simulink model "SF019B_PwrLimr"  (R2013b)
settings: Solver=VariableStepDiscrete  StartTime=0.0  StopTime=10  RelTol=1e-3
values from neighbouring files (symbols this model uses):
  ARCHGLBPRM_2MILLISEC_SEC_F32 = DataDict.Constant    [SF019B_PwrLimr_DataDict.m]
  ELECGLBPRM_IVTRCNT_CNT_U08 = DataDict.ConfigParam    [SF019B_PwrLimr_DataDict.m]
  PwrLimrBackEmfConStdT = DataDict.Calibration    [SF019B_PwrLimr_DataDict.m]
  PwrLimrBrdgVltgAdjSlew = DataDict.Calibration    [SF019B_PwrLimr_DataDict.m]
  PwrLimrBrdgVltgAltFltAdj = DataDict.Calibration    [SF019B_PwrLimr_DataDict.m]
  PwrLimrFilAssiRednThd = DataDict.Calibration    [SF019B_PwrLimr_DataDict.m]
  PwrLimrLoVoltAssiRcvrThd = DataDict.Calibration    [SF019B_PwrLimr_DataDict.m]
  PwrLimrLoVoltAssiRcvrTi = DataDict.Calibration    [SF019B_PwrLimr_DataDict.m]
  PWRLIMRMILLISECTOSEC_SECPERMILLISEC_F32 = DataDict.Constant    [SF019B_PwrLimr_DataDict.m]
  PwrLimrMotEnvlpX = DataDict.Calibration    [SF019B_PwrLimr_DataDict.m]
  PwrLimrMotEnvlpY = DataDict.Calibration    [SF019B_PwrLimr_DataDict.m]
  PwrLimrSpdAdjSlewDec = DataDict.Calibration    [SF019B_PwrLimr_DataDict.m]
  PwrLimrSpdAdjSlewEna = DataDict.Calibration    [SF019B_PwrLimr_DataDict.m]
  PwrLimrSpdAdjSlewInc = DataDict.Calibration    [SF019B_PwrLimr_DataDict.m]
  PwrLimrStdOperMotEnvlpX = DataDict.Calibration    [SF019B_PwrLimr_DataDict.m]
  PwrLimrStdOperMotEnvlpY = DataDict.Calibration    [SF019B_PwrLimr_DataDict.m]
  PwrLimrVltgDptMotVelOffsX = DataDict.Calibration    [SF019B_PwrLimr_DataDict.m]
  PwrLimrVltgDptMotVelOffsY = DataDict.Calibration    [SF019B_PwrLimr_DataDict.m]
undefined symbols (not defined in the file): ARCHGLBPRM_10MILLISEC_SEC_F32, PwrLimrAssiRednLpFilFrq, PwrLimrMotVelLpFilFrq
libraries: simulink x12, NxtrLim x2
(part 2 of 2)

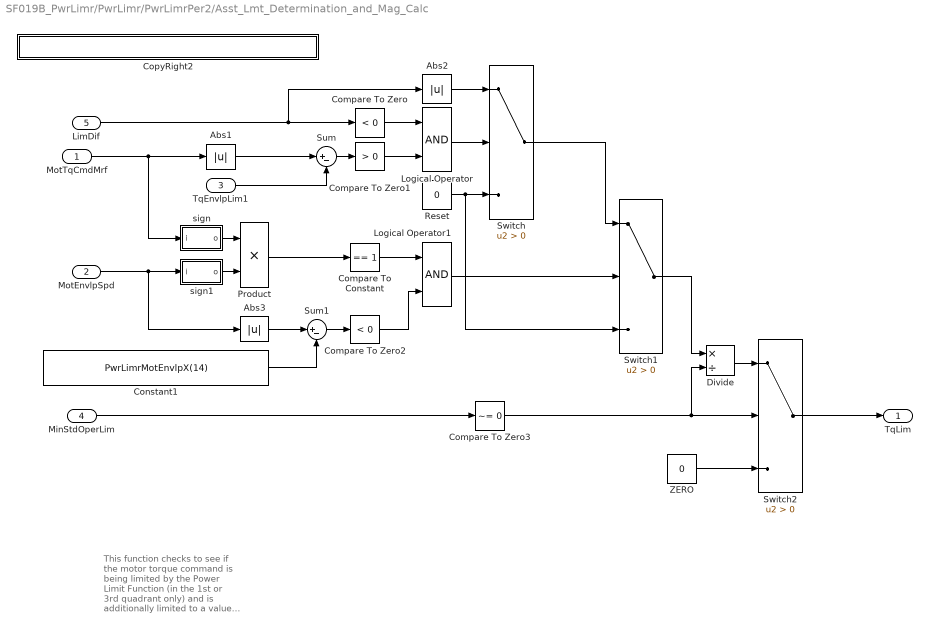
== system SF019B_PwrLimr/PwrLimr/PwrLimrPer2/Asst_Lmt_Determination_and_Mag_Calc ==
  note: This function checks to see if the motor torque command is being limited by the Power Limit Function
      | (in the 1st or 3rd quadrant only) and is additionally limited to a value less than the full performance at
      | the minimum standard operating condition voltage.
      |
      | The magnitude of assist reduction is calculated as the amount of assist reduction divided
      | by full performance in minimum standard operating condition voltage.
  MotTqCmdMrf : Inport
  MotEnvlpSpd : Inport  Port=2
  TqEnvlpLim1 : Inport  Port=3
  MinStdOperLim : Inport  Port=4
  LimDif : Inport  Port=5
  Abs1 : Abs
  Abs2 : Abs
  Abs3 : Abs
  Compare To Constant : simulink/Logic and Bit Operations/Compare To Constant  relop===  const=1  OutDataTypeStr=uint8
  Compare To Zero : simulink/Logic and Bit Operations/Compare To Zero  relop=<  OutDataTypeStr=uint8
  Compare To Zero1 : simulink/Logic and Bit Operations/Compare To Zero  relop=>  OutDataTypeStr=uint8
  Compare To Zero2 : simulink/Logic and Bit Operations/Compare To Zero  relop=<  OutDataTypeStr=uint8
  Compare To Zero3 : simulink/Logic and Bit Operations/Compare To Zero  relop=~=  OutDataTypeStr=uint8
  Constant1 : Constant  Value=PwrLimrMotEnvlpX(14)
  CopyRight2 : Subsystem  Description=|  mask(Copyright Information){none=on}
      | Copyright info block.                                               
      |                                                                     
      | Place copyright information at the top of every subsystem in design.
      mask prompts: none "No parameters"
      mask help: Place copyright information at the top of every subsystem in design.
      mask Display:
      | NxtrConf = 'Nexteer Confidential';
      | 
      | sys = bdroot; %handle for the current model ("system")
      | first = get_param(sys,'Created');
      | first = first(end-3:end);  %year is last four digits
      | 
      | last = get_param(sys,'LastModifiedDate');
      | if isempty(last)
      |     last = datestr(now,'yyyy');
      | else
      |     last = last(end-3:end);
      | end
      | 
      | if strcmp(first,last)
      |     fprintf('%s -- Copyright %s Nexteer',NxtrConf,first)
      | else
      |     fprintf('%s -- %s%s- %s Nexteer',NxtrConf,char(169),first,last)
      | end
  Divide : Product  Inputs=*/
  Logical Operator : Logic  AllPortsSameDT=off  OutDataTypeStr=boolean
  Logical Operator1 : Logic  AllPortsSameDT=off  OutDataTypeStr=boolean
  Product : Product  RndMeth=Zero
  Reset : Constant  Value=0
  Sum : Sum  Inputs=|+-
  Sum1 : Sum  Inputs=|+-
  Switch : Switch  Criteria=u2 > Threshold
  Switch1 : Switch  Criteria=u2 > Threshold
  Switch2 : Switch  Criteria=u2 > Threshold
      settings: AttributesFormatString=Checking for divide-by-zero
  ZERO : Constant  Value=0
  sign : Subsystem  mask(2-state sign){}
      mask help: version: Nov 30, 2012
      mask Help:
      | Input < 0, Output = -1
      | Input = 0, Output = +1
      | Input > 0, Output = +1
      mask Display: disp 'sign'
  sign1 : Subsystem  mask(2-state sign){}
      mask help: version: Nov 30, 2012
      mask Help:
      | Input < 0, Output = -1
      | Input = 0, Output = +1
      | Input > 0, Output = +1
      mask Display: disp 'sign'
  TqLim : Outport
  wires:
  Sum/1 -> Compare To Zero1/1
  Compare To Zero/1 -> Logical Operator/1
  Compare To Zero1/1 -> Logical Operator/2
  Logical Operator/1 -> Switch/2
  Abs2/1 -> Switch/1
  Reset/1 -> Switch/3, Switch1/3
  LimDif/1 -> Compare To Zero/1, Abs2/1
  MotTqCmdMrf/1 -> Abs1/1, sign/1(i)
  TqEnvlpLim1/1 -> Sum/2
  Abs1/1 -> Sum/1
  Switch1/1 -> Divide/1
  MotEnvlpSpd/1 -> Abs3/1, sign1/1(i)
  sign/1(o) -> Product/1
  sign1/1(o) -> Product/2
  Product/1 -> Compare To Constant/1
  Compare To Constant/1 -> Logical Operator1/1
  Switch/1 -> Switch1/1
  Abs3/1 -> Sum1/1
  Constant1/1 -> Sum1/2
  Sum1/1 -> Compare To Zero2/1
  Compare To Zero2/1 -> Logical Operator1/2
  Logical Operator1/1 -> Switch1/2
  MinStdOperLim/1 -> Compare To Zero3/1
  ZERO/1 -> Switch2/3
  Compare To Zero3/1 -> Switch2/2, Divide/2
  Divide/1 -> Switch2/1
  Switch2/1 -> TqLim/1

== system SF019B_PwrLimr/PwrLimr/PwrLimrPer2/CopyRight2 ==

== system SF019B_PwrLimr/PwrLimr/PwrLimrPer1/Battery_Voltage_Fn/CopyRight2 ==

== system SF019B_PwrLimr/PwrLimr/PwrLimrPer1/Max_Mtr_Curr_Lmt_Fn/CopyRight2 ==

== system SF019B_PwrLimr/PwrLimr/PwrLimrPer1/MinStdOp_Volt_Max_Net_Assist/CopyRight2 ==

== system SF019B_PwrLimr/PwrLimr/PwrLimrPer1/OpVel_Offset_Slew_Rate_Lmt/CopyRight2 ==

== system SF019B_PwrLimr/PwrLimr/PwrLimrPer1/Output_Velocity_Fn/Apply_Limit_Else ==
  SignMotEnvlpSpd : Inport
  TqLim1 : Inport  Port=2
  Product2 : Product  RndMeth=Zero
  MRFMtrTrqCmdTemp_MtrNm : Outport
  wires:
  TqLim1/1 -> Product2/2
  SignMotEnvlpSpd/1 -> Product2/1
  Product2/1 -> MRFMtrTrqCmdTemp_MtrNm/1

== system SF019B_PwrLimr/PwrLimr/PwrLimrPer1/Output_Velocity_Fn/Apply_Limit_If ==
  CntDisMtrTrqCmdPerInvMRF : Inport
  SignMotEnvlpSpd : Inport  Port=2
  TqLim1 : Inport  Port=3
  TqLim4 : Inport  Port=4
  Product : Product  RndMeth=Zero
  Product1 : Product  RndMeth=Zero
  Saturation_Dynamic : simulink/Discontinuities/Saturation Dynamic  OutMin=-8.8  OutMax=8.8  OutDataTypeStr=Inherit: Same as second input  OutDataType=fixdt(1, 16)  OutScaling=2^-10  DoSatur=off
  MRFMtrTrqCmdTemp_MtrNm : Outport
  wires:
  Saturation_Dynamic/1 -> Product1/2
  Product/1 -> Saturation_Dynamic/2
  SignMotEnvlpSpd/1 -> Product/1, Product1/1
  TqLim1/1 -> Saturation_Dynamic/1
  Product1/1 -> MRFMtrTrqCmdTemp_MtrNm/1
  CntDisMtrTrqCmdPerInvMRF/1 -> Product/2
  TqLim4/1 -> Saturation_Dynamic/3

== system SF019B_PwrLimr/PwrLimr/PwrLimrPer1/Output_Velocity_Fn/ChooseMax4 ==
  TqEnvlpLim4 : Inport
  TLimMaxCurr : Inport  Port=2
  Gain2 : Gain  Gain=-1
  MinMax3 : MinMax  Function=max  Inputs=2
  TqLim4 : Outport
  wires:
  Gain2/1 -> MinMax3/2
  TqEnvlpLim4/1 -> MinMax3/1
  MinMax3/1 -> TqLim4/1
  TLimMaxCurr/1 -> Gain2/1

== system SF019B_PwrLimr/PwrLimr/PwrLimrPer1/Output_Velocity_Fn/ChooseMin1_Else ==
  TLimMaxCurr : Inport
  TqEnvlpLim1 : Inport  Port=2
  MinMax2 : MinMax  Inputs=2
  TqLim1 : Outport
  wires:
  TqEnvlpLim1/1 -> MinMax2/2
  TLimMaxCurr/1 -> MinMax2/1
  MinMax2/1 -> TqLim1/1

== system SF019B_PwrLimr/PwrLimr/PwrLimrPer1/Output_Velocity_Fn/ChooseMin1_If ==
  TLimMaxCurr : Inport
  TqEnvlpLim1 : Inport  Port=2
  MinMax2 : MinMax  Inputs=2
  TqLim1 : Outport
  wires:
  MinMax2/1 -> TqLim1/1
  TLimMaxCurr/1 -> MinMax2/1
  TqEnvlpLim1/1 -> MinMax2/2

== system SF019B_PwrLimr/PwrLimr/PwrLimrPer1/Output_Velocity_Fn/CopyRight2 ==

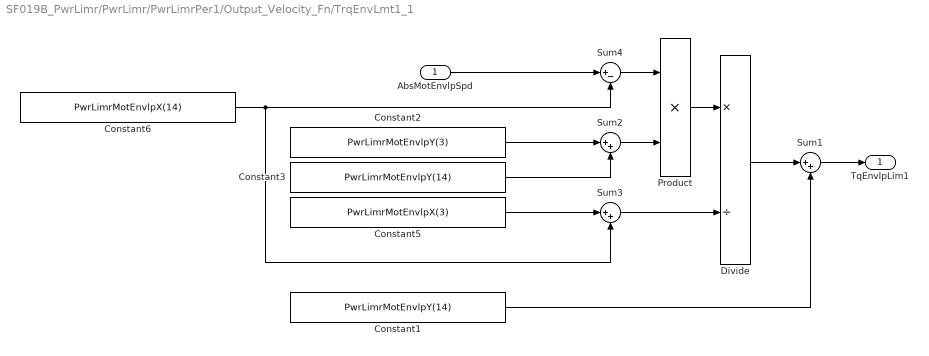
== system SF019B_PwrLimr/PwrLimr/PwrLimrPer1/Output_Velocity_Fn/TrqEnvLmt1_1 ==
  AbsMotEnvlpSpd : Inport
  Constant1 : Constant  Value=PwrLimrMotEnvlpY(14)
  Constant2 : Constant  Value=PwrLimrMotEnvlpY(3)
  Constant3 : Constant  Value=PwrLimrMotEnvlpY(14)
  Constant5 : Constant  Value=PwrLimrMotEnvlpX(3)
  Constant6 : Constant  Value=PwrLimrMotEnvlpX(14)
  Divide : Product  Inputs=*/
  Product : Product  RndMeth=Zero
  Sum1 : Sum  Inputs=|++
  Sum2 : Sum  Inputs=|++
  Sum3 : Sum  Inputs=|++
  Sum4 : Sum  Inputs=|+-
  TqEnvlpLim1 : Outport
  wires:
  Constant5/1 -> Sum3/1
  Constant3/1 -> Sum2/2
  Divide/1 -> Sum1/1
  Constant2/1 -> Sum2/1
  Constant6/1 -> Sum3/2, Sum4/2
  AbsMotEnvlpSpd/1 -> Sum4/1
  Sum3/1 -> Divide/2
  Product/1 -> Divide/1
  Sum2/1 -> Product/2
  Sum4/1 -> Product/1
  Constant1/1 -> Sum1/2
  Sum1/1 -> TqEnvlpLim1/1

== system SF019B_PwrLimr/PwrLimr/PwrLimrPer1/Output_Velocity_Fn/TrqEnvLmt1_2 ==
  AbsMotEnvlpSpd : Inport
  TrqEnvTbl : Lookup  InputValues=PwrLimrMotEnvlpX  Table=PwrLimrMotEnvlpY  LookUpMeth=Interpolation-Use End Values
      settings: AttributesFormatString=%<InputValues>\n%<Table>
  TqEnvlpLim1 : Outport
  wires:
  AbsMotEnvlpSpd/1 -> TrqEnvTbl/1
  TrqEnvTbl/1 -> TqEnvlpLim1/1

== system SF019B_PwrLimr/PwrLimr/PwrLimrPer1/Output_Velocity_Fn/TrqEnvLmt4 ==
  AbsMotEnvlpSpd : Inport
  Gain : Gain  Gain=-1
  Gain1 : Gain  Gain=-1
  TrqEnvTbl_ : Lookup  InputValues=PwrLimrMotEnvlpX  Table=PwrLimrMotEnvlpY  LookUpMeth=Interpolation-Use End Values
      settings: AttributesFormatString=%<InputValues>\n%<Table>
  TqEnvlpLim4 : Outport
  wires:
  Gain1/1 -> TrqEnvTbl_/1
  TrqEnvTbl_/1 -> Gain/1
  AbsMotEnvlpSpd/1 -> Gain1/1
  Gain/1 -> TqEnvlpLim4/1

== system SF019B_PwrLimr/PwrLimr/PwrLimrPer1/Output_Velocity_Fn/sign ==
  note: REVISIONS
      |   Jan 31, 2012.  Date created.
      |   Nov 30, 2012.  Edited mask because block was taking up too much space when placed into models.
  note: Simulink Sign block has three states (-1, 0, +1)
      | This block defines zero input as +1 sign.
  i : Inport
  Constant : Constant
  Constant1 : Constant  Value=-1
  Switch2 : Switch
  o : Outport
  wires:
  Constant/1 -> Switch2/1
  Constant1/1 -> Switch2/3
  i/1 -> Switch2/2
  Switch2/1 -> o/1

== system SF019B_PwrLimr/PwrLimr/PwrLimrPer1/TrqCmd_Scl_Inverter/CopyRight2 ==

== system SF019B_PwrLimr/PwrLimr/PwrLimrPer2/AssiLimMgnFil/1LP1-CF Filter ==
  note: REVISIONS
      |   Feb 13, 2012.  Date created.
      |   Feb 17, 2012.  Conversion from Hz to Knum moved to Initialization tab of mask dialog box.
      |   Feb 20, 2012.  Parameterized 1/z block Initial Condition instead of hard-coded = 0.
      |   Jun 14, 2012.  Edited Icon to match other 1LP1-CF variants.
  note: This Subsystem represents a type 1LP1-CF Low-Pass filter with floating point math. Layout and nomenclature taken from Design Document authored by Mark Colosky.
  note: Filter layout from spreadsheet
  In1 : Inport
  Constant : Constant  Value=Knum
  Integer Delay : Delay  DelayLength=1  InitialCondition=IC
  Product1 : Product  RndMeth=Zero
  Sum : Sum  Inputs=|+-
  Sum1 : Sum  Inputs=|++
  Out : Outport
  wires:
  Sum/1 -> Product1/2  "c"
  Constant/1 -> Product1/1
  Product1/1 -> Sum1/1  "d"
  Integer Delay/1 -> Sum1/2, Sum/2  "f"
  In1/1 -> Sum/1  "Unfiltered_Signal"
  Sum1/1 -> Integer Delay/1, Out/1  "e"

== system SF019B_PwrLimr/PwrLimr/PwrLimrPer2/AssiLimMgnFil/CopyRight2 ==

== system SF019B_PwrLimr/PwrLimr/PwrLimrPer2/Asst_Lmt_Condition_Determination/CopyRight2 ==

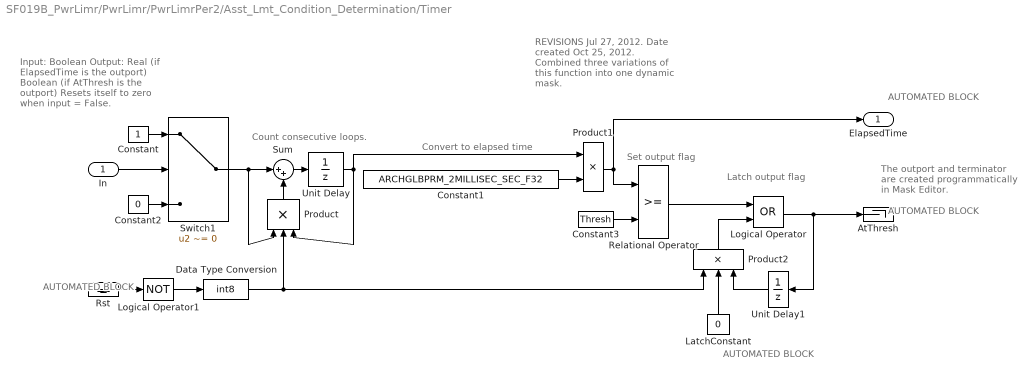
== system SF019B_PwrLimr/PwrLimr/PwrLimrPer2/Asst_Lmt_Condition_Determination/Timer ==
  note: Input:  Boolean
      | Output:  Real (if ElapsedTime is the outport)
      |                Boolean (if AtThresh is the outport)
      |
      | Resets itself to zero when input = False.
  note: REVISIONS
      |   Jul 27, 2012.  Date created
      |   Oct 25, 2012. Combined three variations of this function into one dynamic mask.
  note: Count consecutive loops.
  note: Convert to elapsed time
  note: The outport and terminator are created
      | programmatically in Mask Editor.
  note: AUTOMATED BLOCK
  note: AUTOMATED BLOCK
  note: AUTOMATED BLOCK
  note: AUTOMATED BLOCK
  note: Set output flag
  note: Latch output flag
  In : Inport
  AtThresh : Terminator
  Constant : Constant
  Constant1 : Constant  Value=ARCHGLBPRM_2MILLISEC_SEC_F32
  Constant2 : Constant  Value=0
  Constant3 : Constant  Value=Thresh
  Data Type Conversion : DataTypeConversion  OutDataTypeStr=int8
  LatchConstant : Constant  Value=0
  Logical Operator : Logic  Operator=OR  AllPortsSameDT=off  OutDataTypeStr=boolean
  Logical Operator1 : Logic  Operator=NOT  AllPortsSameDT=off  OutDataTypeStr=boolean
  Product : Product  Inputs=3  RndMeth=Zero
  Product1 : Product  RndMeth=Zero
  Product2 : Product  Inputs=3  RndMeth=Zero
  Relational Operator : RelationalOperator  OutDataTypeStr=boolean
  Rst : Ground
  Sum : Sum  Inputs=|++
  Switch1 : Switch  Criteria=u2 ~= 0  Threshold=0.5  OutDataTypeStr=double  InputSameDT=on
  Unit Delay : UnitDelay  SampleTime=-1
  Unit Delay1 : UnitDelay  SampleTime=-1
  ElapsedTime : Outport
  wires:
  Constant/1 -> Switch1/1
  Constant2/1 -> Switch1/3
  Switch1/1 -> Sum/1, Product/1
  Sum/1 -> Unit Delay/1
  Unit Delay/1 -> Product1/1, Product/3
  Product/1 -> Sum/2
  In/1 -> Switch1/2
  Product1/1 -> Relational Operator/1, ElapsedTime/1
  Constant1/1 -> Product1/2
  Constant3/1 -> Relational Operator/2
  Product2/1 -> Logical Operator/2
  Data Type Conversion/1 -> Product2/1, Product/2
  Rst/1 -> Logical Operator1/1
  Logical Operator/1 -> AtThresh/1, Unit Delay1/1
  Relational Operator/1 -> Logical Operator/1
  Unit Delay1/1 -> Product2/3
  LatchConstant/1 -> Product2/2
  Logical Operator1/1 -> Data Type Conversion/1

== system SF019B_PwrLimr/PwrLimr/PwrLimrPer2/Asst_Lmt_Determination_and_Mag_Calc/CopyRight2 ==

== system SF019B_PwrLimr/PwrLimr/PwrLimrPer2/Asst_Lmt_Determination_and_Mag_Calc/sign ==
  note: REVISIONS
      |   Jan 31, 2012.  Date created.
      |   Nov 30, 2012.  Edited mask because block was taking up too much space when placed into models.
  note: Simulink Sign block has three states (-1, 0, +1)
      | This block defines zero input as +1 sign.
  i : Inport
  Constant : Constant
  Constant1 : Constant  Value=-1
  Switch2 : Switch
  o : Outport
  wires:
  Constant/1 -> Switch2/1
  Constant1/1 -> Switch2/3
  i/1 -> Switch2/2
  Switch2/1 -> o/1

== system SF019B_PwrLimr/PwrLimr/PwrLimrPer2/Asst_Lmt_Determination_and_Mag_Calc/sign1 ==
  note: Simulink Sign block has three states (-1, 0, +1)
      | This block defines zero input as +1 sign.
  note: REVISIONS
      |   Jan 31, 2012.  Date created.
      |   Nov 30, 2012.  Edited mask because block was taking up too much space when placed into models.
  i : Inport
  Constant : Constant
  Constant1 : Constant  Value=-1
  Switch2 : Switch
  o : Outport
  wires:
  Switch2/1 -> o/1
  i/1 -> Switch2/2
  Constant1/1 -> Switch2/3
  Constant/1 -> Switch2/1
